simulink model "Powertrain_Performance_Design"  (R2024a)
settings: Solver=ode4  StartTime=0.0  StopTime=simtime  FixedStep=1  MaxStep=0.1  RelTol=1e-3
model workspace (MAT data in the model file):
  A_max = 2.22
  C_d = 0.23
  C_r = 0.011
  Cpack = 216
  DOD = [0 0.1 0.2 0.3 0.4 0.5 0.6 0.7 0.8 0.9 1 1.1 ... (1001 elements, 1001x1)]
  EM_N = [0 100 200 300 400 500 600 700 800 900 1000 1100 1200 1300 1400 1500 1600 1700 1800 1900 2000 2100 2200 2300 2400 2500 2600 2700 2800 2900 3000 3100 3200 3300 3400 3500 3600 3700 3800 3900 4000 4100 4200 4300 4400 4500 4600 4700 4800 4900 5000 5100 5200 5300 5400 5500 5600 5700 5800 5900 6000 6100 6200 6300 6400 6500 6600 6700 6800 6900 7000 7100 7200 7300 7400 7500 7600 7700 7800 7900 8000 8100 8200 8300 8400 8500 8600 8700 8800 8900 9000 9100 9200 9300 9400 9500 9600 9700 9800 9900 10000 10100 10200 10300 10400 10500 10600 10700 10800 10900 11000 11100 11200 11300 11400 11500 11600 11700 11800 11900 12000 12100 12200 12300 12400 12500 12600 12700 12800 12900 13000 13100 13200 13300 13400 13500 13600 13700 13800 13900 14000 14100 14200 14300 14400 14500 14600 14700 14800 14900 15000 15100 15200 15300 15400 15500 15600 15700 15800 15900 16000 16100 16200 16300 16400 16500 16600 16700 16800 16900 17000]
  EM_N_Max = 17000
  EM_N_Min = 0
  EM_eff = Simulink.Parameter
  EM_eff.Value = [78 78 78 78 78 78 78 78 78 78 78 78 ... (250000 elements, 500x500)]
  EM_eff.Complexity = 'real'
  EM_eff.Dimensions = [500 500]
  EM_eff.DataType = 'auto'
  Ff_N = 10218
  Kd = 0.3
  Ki = 0.02
  Kp = 15
  N_EM_eff = [0 34.06813627 68.13627255 102.2044088 136.2725451 170.3406814 204.4088176 238.4769539 272.5450902 306.6132265 340.6813627 374.749499 ... (500 elements, 1x500)]
  T_EM_Cont = [181.43664; 181.43664; 181.43664; 181.43664; 181.43664; 181.43664; 181.43664; 181.43664; 181.43664; 181.43664; 181.43664; 181.43664; 181.43664; 181.43664; 181.43664; 181.43664; 181.43664; 181.43664; 181.43664; 181.43664; 181.43664; 181.43664; 181.43664; 181.43664; 181.43664; 181.43664; 181.43664; 181.43664; 181.43664; 181.43664; 181.43664; 181.43664; 181.43664; 181.43664; 181.43664; 181.43664; 181.43664; 181.43664; 181.43664; 181.43664; 181.43664; 181.43664; 181.43664; 181.43664; 181.43664; 181.43664; 181.43664; 181.43664; 181.43664; 181.43664; 181.43664; 177.87905; 174.4583; 171.16664; 167.99688; 164.9424; 161.997; 159.15494; 156.41089; 153.75986; 151.1972; 148.71855; 146.31987; 143.99733; 141.74737; 139.56664; 137.452; 135.40047; 133.40929; 131.47582; 129.5976; 127.77228; 125.99766; 124.27167; 122.59232; 120.95776; 119.36621; 117.816; 116.30554; 114.83331; 113.3979; 111.99792; 110.63209; 109.29918; 107.998; 106.72743; 105.48642; 104.27393; 103.089; 101.93069; 100.79813; 99.690459; 98.606867; 97.546578; 96.508848; 95.492966; 94.498247; 93.524039; 92.569712; 91.634664; 90.718318; 89.820116; 88.939527; 88.076036; 87.229152; 86.398398; 85.583318; 84.783474; 83.998442; 83.227814; 82.471198; 81.728214; 80.998498; 80.281697; 79.577472; 78.885494; 78.205446; 77.537024; 76.87993; 76.23388; 75.598598; 74.973816; 74.359277; 73.75473; 73.159934; 72.574654; 71.998665; 71.431746; 70.873686; 70.324277; 69.783321; 69.250624; 68.725998; 68.209261; 67.700237; 67.198754; 66.704645; 66.21775; 65.737911; 65.264977; 64.798798; 64.339232; 63.886139; 63.439383; 62.998832; 62.564357; 62.135834; 61.713141; 61.296161; 60.884777; 60.478878; 60.078356; 59.683104; 59.293018; 58.907998; 58.527947; 58.152768; 57.782368; 57.416657; 57.055546; 56.698948; 56.346781; 55.998961; 55.65541; 55.316047; 54.980799; 54.649589; 54.322346; 53.998999; 53.679478; 53.363716]
  T_EM_Max = 375
  T_EM_Min = -375
  T_EM_Peak = [375; 375; 375; 375; 375; 375; 375; 375; 375; 375; 375; 375; 375; 375; 375; 375; 375; 375; 375; 375; 375; 375; 375; 375; 375; 375; 375; 375; 375; 375; 375; 375; 375; 375; 375; 375; 375; 375; 375; 375; 375; 375; 375; 375; 375; 375; 375; 375; 375; 375; 375; 368.86499; 361.77143; 354.94555; 348.37249; 342.03844; 335.93061; 330.03709; 324.3468; 318.84939; 313.53524; 308.39532; 303.4212; 298.60499; 293.93929; 289.41714; 285.03203; 280.77782; 276.64874; 272.63934; 268.74449; 264.95936; 261.27936; 257.7002; 254.21776; 250.82819; 247.52782; 244.31317; 241.18095; 238.12803; 235.15143; 232.24832; 229.41603; 226.65198; 223.95374; 221.31899; 218.74551; 216.2312; 213.77403; 211.37207; 209.02349; 206.72653; 204.4795; 202.2808; 200.12888; 198.02226; 195.95952; 193.93932; 191.96035; 190.02136; 188.12114; 186.25856; 184.43249; 182.64189; 180.88571; 179.16299; 177.47278; 175.81415; 174.18624; 172.5882; 171.01922; 169.47851; 167.96531; 166.47889; 165.01855; 163.5836; 162.1734; 160.7873; 159.4247; 158.08499; 156.76762; 155.47202; 154.19766; 152.94402; 151.7106; 150.49691; 149.30249; 148.12688; 146.96964; 145.83034; 144.70857; 143.60393; 142.51602; 141.44447; 140.38891; 139.34899; 138.32437; 137.3147; 136.31967; 135.33895; 134.37224; 133.41925; 132.47968; 131.55325; 130.63968; 129.73872; 128.8501; 127.97357; 127.10888; 126.2558; 125.4141; 124.58354; 123.76391; 122.955; 122.15659; 121.36848; 120.59048; 119.82238; 119.06401; 118.31518; 117.57571; 116.84543; 116.12416; 115.41174; 114.70801; 114.01281; 113.32599; 112.64739; 111.97687; 111.31429; 110.6595]
  Tq_EM_eff = [0 0.751503006 1.503006012 2.254509018 3.006012024 3.75751503 4.509018036 5.260521042 6.012024048 6.763527054 7.51503006 8.266533066 ... (500 elements, 1x500)]
  Upack = [405.9 404.506 403.17334 401.89932 400.68136 399.51699 398.40386 397.33971 396.32239 395.34983 394.42006 393.53121 ... (1001 elements, 1001x1)]
  Upack_max = 405.9
  Vmax = 250
  a_r = 1.202
  eta_pack = 0.97
  eta_tr = 0.95
  g = 9.81
  ix = 9
  lambda_m = 1.05
  m_v = 1862
  r_w = 0.3277
  t_cool = 250
  t_peak = 20
values from neighbouring files (symbols this model uses):
  EM_eff = [78 78 78 78 78 78 78 78 78 78 78 78 ... (250000 elements, 500x500)]    [EM_eff.mat]
undefined symbols (not defined in the file or in its folder): selection, Soc_init, theta
(part 1 of 2)
settings Model: Creator=Kimo Store  LastModifiedBy=Kimo Store
settings DataIOCC: SaveOutput=off  ReturnWorkspaceOutputs=off  LoggingToFile=on
settings ConfigComp: DVTestSuiteOptimization=Auto  DVDetectOutOfBounds=on  DVModelReferenceHarness=on  DVHarnessSource=Signal Editor

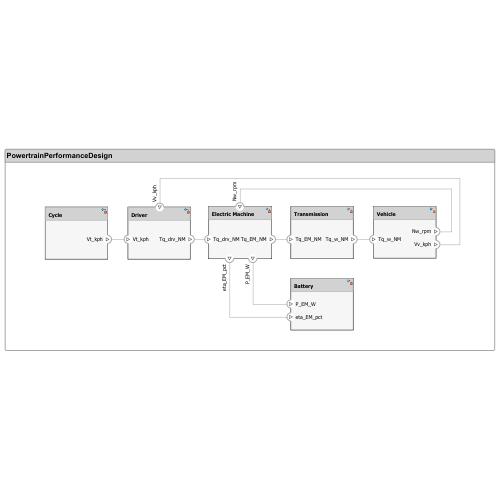
[thumbnail: Simulink's stored preview of the top-level diagram]
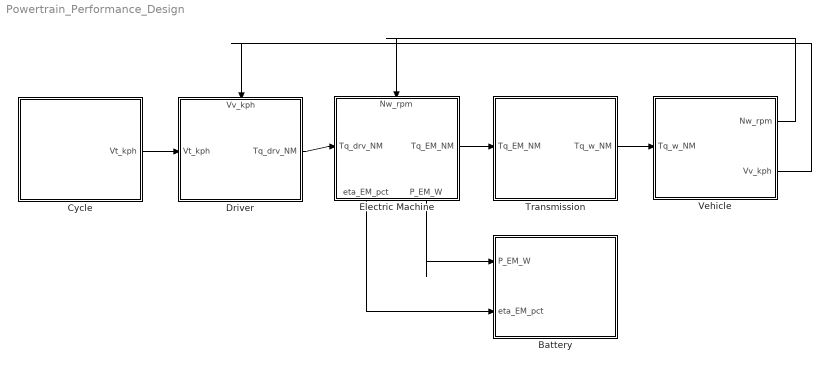
== system Powertrain_Performance_Design ==
  Battery : Subsystem
      settings: PortSchema="{\"entries\":[{\"content\":{\"headerSize\":26,\"margin\":15,\"minimumSpacing\":25,\"sides\":[{\"content\":{\"connectorIds\":[\"In1\",\"In2\"]},\"type\":\"ConnectorPlacement.EquallySpacedRectSide\",\"uuid\":\"68db000f-08f3-43d6-8df8-ef1e265f9696\"},{\"content\":{\"side\":\"RIGHT\"},\"type\":\"ConnectorPlacement.EquallySpacedRectSide\",\"uuid\":\"83cc5010-d255-45a5-b8a1-63c53c107bd8\"},{\"content\":{\"side\":\"TOP\"},\"type\":\"ConnectorPlacement.EquallySpacedRectSide\",\"uuid\":\"8183809d-813b-433e-980f-1f031c5b719a\"}]},\"type\":\"ConnectorPlacement.EquallySpacedConnector\",\"uuid\":\"7d483e94-2e91-4ff8-9657-91e4b1686e41\"}],\"packageUris\":[\"http://schema.mathworks.com/mf0/Connector/R2020b\"],\"version\":\"1.0\"}"
  Cycle : Subsystem
      settings: PortSchema="{\"entries\":[{\"content\":{\"headerSize\":26,\"margin\":15,\"minimumSpacing\":25,\"sides\":[{\"content\":{},\"type\":\"ConnectorPlacement.EquallySpacedRectSide\",\"uuid\":\"68db000f-08f3-43d6-8df8-ef1e265f9696\"},{\"content\":{\"connectorIds\":[\"Out1\"],\"side\":\"RIGHT\"},\"type\":\"ConnectorPlacement.EquallySpacedRectSide\",\"uuid\":\"83cc5010-d255-45a5-b8a1-63c53c107bd8\"},{\"content\":{\"side\":\"TOP\"},\"type\":\"ConnectorPlacement.EquallySpacedRectSide\",\"uuid\":\"8183809d-813b-433e-980f-1f031c5b719a\"}]},\"type\":\"ConnectorPlacement.EquallySpacedConnector\",\"uuid\":\"7d483e94-2e91-4ff8-9657-91e4b1686e41\"}],\"packageUris\":[\"http://schema.mathworks.com/mf0/Connector/R2020b\"],\"version\":\"1.0\"}"
  Driver : Subsystem
      settings: PortSchema="{\"entries\":[{\"content\":{\"headerSize\":26,\"margin\":15,\"minimumSpacing\":25,\"sides\":[{\"content\":{\"connectorIds\":[\"In2\"]},\"type\":\"ConnectorPlacement.EquallySpacedRectSide\",\"uuid\":\"68db000f-08f3-43d6-8df8-ef1e265f9696\"},{\"content\":{\"connectorIds\":[\"Out1\"],\"side\":\"RIGHT\"},\"type\":\"ConnectorPlacement.EquallySpacedRectSide\",\"uuid\":\"83cc5010-d255-45a5-b8a1-63c53c107bd8\"},{\"content\":{\"connectorIds\":[\"In1\"],\"side\":\"TOP\"},\"type\":\"ConnectorPlacement.EquallySpacedRectSide\",\"uuid\":\"8183809d-813b-433e-980f-1f031c5b719a\"}]},\"type\":\"ConnectorPlacement.EquallySpacedConnector\",\"uuid\":\"7d483e94-2e91-4ff8-9657-91e4b1686e41\"}],\"packageUris\":[\"http://schema.mathworks.com/mf0/Connector/R2020b\"],\"version\":\"1.0\"}"
  Electric Machine : Subsystem
      settings: PortSchema="{\"entries\":[{\"content\":{\"headerSize\":26,\"margin\":15,\"minimumSpacing\":25,\"sides\":[{\"content\":{\"connectorIds\":[\"In2\"]},\"type\":\"ConnectorPlacement.EquallySpacedRectSide\",\"uuid\":\"68db000f-08f3-43d6-8df8-ef1e265f9696\"},{\"content\":{\"connectorIds\":[\"Out1\"],\"side\":\"RIGHT\"},\"type\":\"ConnectorPlacement.EquallySpacedRectSide\",\"uuid\":\"83cc5010-d255-45a5-b8a1-63c53c107bd8\"},{\"content\":{\"connectorIds\":[\"In1\"],\"side\":\"TOP\"},\"type\":\"ConnectorPlacement.EquallySpacedRectSide\",\"uuid\":\"8183809d-813b-433e-980f-1f031c5b719a\"},{\"content\":{\"connectorIds\":[\"Out3\",\"Out2\"],\"side\":\"BOTTOM\"},\"type\":\"ConnectorPlacement.EquallySpacedRectSide\",\"uuid\":\"47240857-0798-46c4-9ad5-1efcb742b832\"}]},\"type\":\"ConnectorPlacement.EquallySpacedConnector\",\"uuid\":\"7d483e94-2e91-4ff8-9657-91e4b1686e41\"}],\"packageUris\":[\"http://schema.mathworks.com/mf0/Connector/R2020b\"],\"version\":\"1.0\"}"
  Transmission : Subsystem
      settings: PortSchema="{\"entries\":[{\"content\":{\"headerSize\":26,\"margin\":15,\"minimumSpacing\":25,\"sides\":[{\"content\":{\"connectorIds\":[\"In1\"]},\"type\":\"ConnectorPlacement.EquallySpacedRectSide\",\"uuid\":\"68db000f-08f3-43d6-8df8-ef1e265f9696\"},{\"content\":{\"connectorIds\":[\"Out1\"],\"side\":\"RIGHT\"},\"type\":\"ConnectorPlacement.EquallySpacedRectSide\",\"uuid\":\"83cc5010-d255-45a5-b8a1-63c53c107bd8\"},{\"content\":{\"side\":\"TOP\"},\"type\":\"ConnectorPlacement.EquallySpacedRectSide\",\"uuid\":\"8183809d-813b-433e-980f-1f031c5b719a\"}]},\"type\":\"ConnectorPlacement.EquallySpacedConnector\",\"uuid\":\"7d483e94-2e91-4ff8-9657-91e4b1686e41\"}],\"packageUris\":[\"http://schema.mathworks.com/mf0/Connector/R2020b\"],\"version\":\"1.0\"}"
  Vehicle : Subsystem
      settings: PortSchema="{\"entries\":[{\"content\":{\"headerSize\":26,\"margin\":15,\"minimumSpacing\":25,\"sides\":[{\"content\":{\"connectorIds\":[\"In1\"]},\"type\":\"ConnectorPlacement.EquallySpacedRectSide\",\"uuid\":\"68db000f-08f3-43d6-8df8-ef1e265f9696\"},{\"content\":{\"connectorIds\":[\"Out1\",\"Out2\"],\"side\":\"RIGHT\"},\"type\":\"ConnectorPlacement.EquallySpacedRectSide\",\"uuid\":\"83cc5010-d255-45a5-b8a1-63c53c107bd8\"},{\"content\":{\"side\":\"TOP\"},\"type\":\"ConnectorPlacement.EquallySpacedRectSide\",\"uuid\":\"8183809d-813b-433e-980f-1f031c5b719a\"},{\"content\":{\"side\":\"BOTTOM\"},\"type\":\"ConnectorPlacement.EquallySpacedRectSide\",\"uuid\":\"d8f33a88-2120-49d7-a1ee-2682923ccda4\"}]},\"type\":\"ConnectorPlacement.EquallySpacedConnector\",\"uuid\":\"7d483e94-2e91-4ff8-9657-91e4b1686e41\"}],\"packageUris\":[\"http://schema.mathworks.com/mf0/Connector/R2020b\"],\"version\":\"1.0\"}"
  wires:
  Electric Machine/2(P_EM_W) -> Battery/1(P_EM_W)
  Driver/1(Tq_drv_NM) -> Electric Machine/2(Tq_drv_NM)
  Vehicle/1(Nw_rpm) -> Electric Machine/1(Nw_rpm)
  Transmission/1(Tq_w_NM) -> Vehicle/1(Tq_w_NM)
  Electric Machine/3(eta_EM_pct) -> Battery/2(eta_EM_pct)
  Electric Machine/1(Tq_EM_NM) -> Transmission/1(Tq_EM_NM)
  Vehicle/2(Vv_kph) -> Driver/1(Vv_kph)
  Cycle/1(Vt_kph) -> Driver/2(Vt_kph)

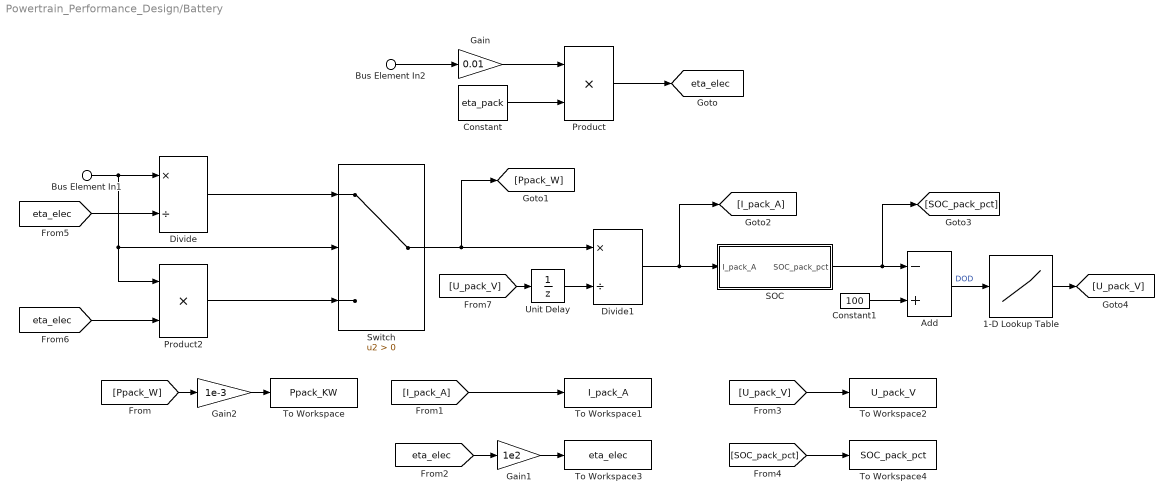
== system Powertrain_Performance_Design/Battery ==
  Bus Element In1 : Inport  PortName=P_EM_W
  Bus Element In2 : Inport  Port=2  PortName=eta_EM_pct
  1-D Lookup Table : Lookup_n-D  NumberOfTableDimensions=1  BreakpointsForDimension1=DOD  Table=Upack  InternalRulePriority=Speed  RndMeth=Simplest
  Add : Sum  Inputs=-+
  Constant : Constant  Value=eta_pack
  Constant1 : Constant  Value=100
  Divide : Product  Inputs=*/
  Divide1 : Product  Inputs=*/
  Gain : Gain  Gain=0.01
  Gain1 : Gain  Gain=1e2
  Gain2 : Gain  Gain=1e-3
  Product : Product
  Product2 : Product
  SOC : Subsystem
  Switch : Switch  Criteria=u2 > Threshold  SaturateOnIntegerOverflow=off  InputSameDT=off
  To Workspace : ToWorkspace  VariableName=Ppack_KW  SaveFormat=Timeseries  SampleTime=-1
  To Workspace1 : ToWorkspace  VariableName=I_pack_A  SaveFormat=Timeseries  SampleTime=-1
  To Workspace2 : ToWorkspace  VariableName=U_pack_V  SaveFormat=Timeseries  SampleTime=-1
  To Workspace3 : ToWorkspace  VariableName=eta_elec  SaveFormat=Timeseries  SampleTime=-1
  To Workspace4 : ToWorkspace  VariableName=SOC_pack_pct  SaveFormat=Timeseries  SampleTime=-1
  Unit Delay : UnitDelay  InitialCondition=405.9  SampleTime=-1  HasFrameUpgradeWarning=on
  tag scope: eta_elec=global
  wires:
  Bus Element In2/1 -> Gain/1
  Gain/1 -> Product/1
  Constant/1 -> Product/2
  Product/1 -> [eta_elec]
  [Ppack_W] -> Gain2/1
  [I_pack_A] -> To Workspace1/1
  [U_pack_V] -> To Workspace2/1
  [SOC_pack_pct] -> To Workspace4/1
  [eta_elec] -> Gain1/1
  Gain1/1 -> To Workspace3/1
  Divide/1 -> Switch/1
  Product2/1 -> Switch/3
  Switch/1 -> Divide1/1, [Ppack_W]
  Bus Element In1/1 -> Switch/2, Product2/1, Divide/1
  [eta_elec] -> Divide/2
  [eta_elec] -> Product2/2
  Divide1/1 -> [I_pack_A], SOC/1(I_pack_A)
  SOC/1(SOC_pack_pct) -> [SOC_pack_pct], Add/1
  Constant1/1 -> Add/2
  Unit Delay/1 -> Divide1/2
  [U_pack_V] -> Unit Delay/1
  Add/1 -> 1-D Lookup Table/1  "DOD"
  1-D Lookup Table/1 -> [U_pack_V]
  Gain2/1 -> To Workspace/1

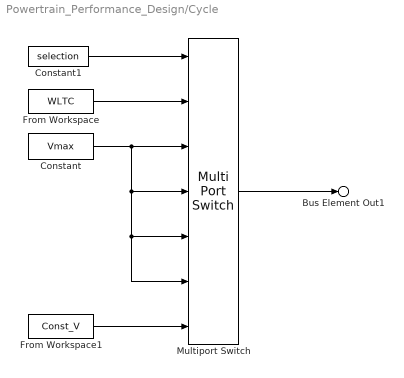
== system Powertrain_Performance_Design/Cycle ==
  Constant : Constant  Value=Vmax
  Constant1 : Constant  Value=selection
  From Workspace : FromWorkspace  VariableName=WLTC
  From Workspace1 : FromWorkspace  VariableName=Const_V
  Multiport Switch : MultiPortSwitch  Inputs=6  SaturateOnIntegerOverflow=off  InputSameDT=off
  Bus Element Out1 : Outport  PortName=Vt_kph
  wires:
  Multiport Switch/1 -> Bus Element Out1/1
  From Workspace/1 -> Multiport Switch/2
  Constant/1 -> Multiport Switch/5, Multiport Switch/6, Multiport Switch/4, Multiport Switch/3
  Constant1/1 -> Multiport Switch/1
  From Workspace1/1 -> Multiport Switch/7

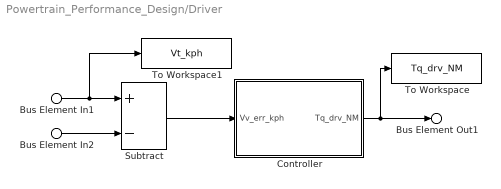
== system Powertrain_Performance_Design/Driver ==
  Bus Element In2 : Inport  PortName=Vv_kph
  Bus Element In1 : Inport  Port=2  PortName=Vt_kph
  Controller : Subsystem
  Subtract : Sum  Inputs=+-
  To Workspace : ToWorkspace  VariableName=Tq_drv_NM  SaveFormat=Timeseries  SampleTime=-1
  To Workspace1 : ToWorkspace  VariableName=Vt_kph  SaveFormat=Timeseries  SampleTime=-1
  Bus Element Out1 : Outport  PortName=Tq_drv_NM
  wires:
  Bus Element In1/1 -> To Workspace1/1, Subtract/1
  Bus Element In2/1 -> Subtract/2
  Subtract/1 -> Controller/1(Vv_err_kph)
  Controller/1(Tq_drv_NM) -> To Workspace/1, Bus Element Out1/1

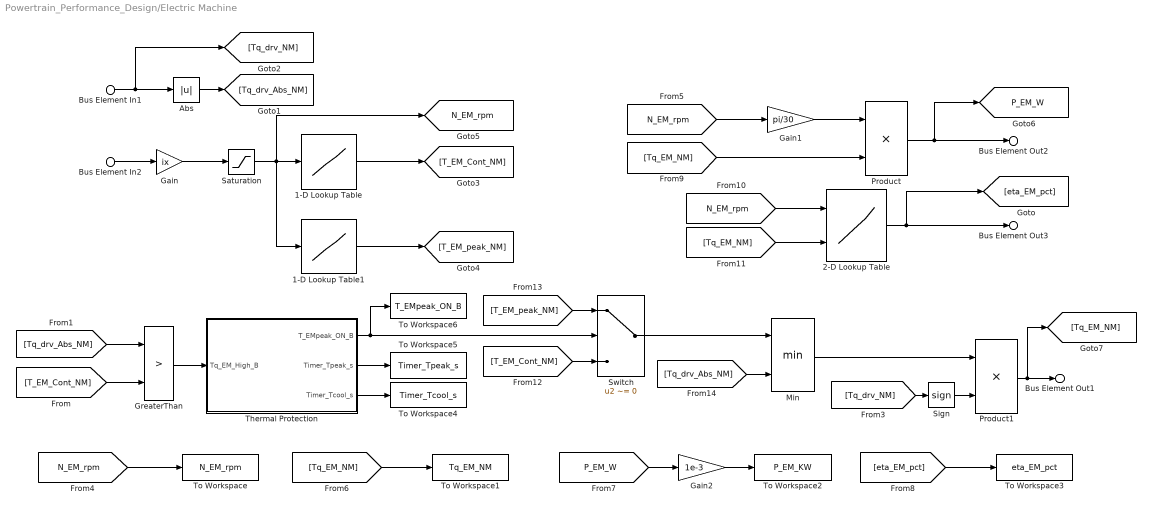
== system Powertrain_Performance_Design/Electric Machine ==
  Bus Element In2 : Inport  PortName=Nw_rpm
  Bus Element In1 : Inport  Port=2  PortName=Tq_drv_NM
  1-D Lookup Table : Lookup_n-D  NumberOfTableDimensions=1  BreakpointsForDimension1=EM_N  Table=T_EM_Cont  InternalRulePriority=Speed  RndMeth=Simplest
  1-D Lookup Table1 : Lookup_n-D  NumberOfTableDimensions=1  BreakpointsForDimension1=EM_N  Table=T_EM_Peak  InternalRulePriority=Speed  RndMeth=Simplest
  2-D Lookup Table : Lookup_n-D  BreakpointsForDimension1=N_EM_eff  BreakpointsForDimension2=Tq_EM_eff  Table=EM_eff  InternalRulePriority=Speed  RndMeth=Simplest
      settings: InputPortMap=u0,u1
  Abs : Abs  SaturateOnIntegerOverflow=off
  Gain : Gain  Gain=ix
  Gain1 : Gain  Gain=pi/30
  Gain2 : Gain  Gain=1e-3
  GreaterThan : RelationalOperator  Operator=>  OutDataTypeStr=boolean  RndMeth=Simplest  InputSameDT=off
  Min : MinMax  Inputs=2
  Product : Product
  Product1 : Product
  Saturation : Saturate  UpperLimit=EM_N_Max  LowerLimit=EM_N_Min
  Sign : Signum
  Switch : Switch  Criteria=u2 ~= 0  SaturateOnIntegerOverflow=off  InputSameDT=off
  Thermal Protection : Subsystem
  To Workspace : ToWorkspace  VariableName=N_EM_rpm  SaveFormat=Timeseries  SampleTime=-1
  To Workspace1 : ToWorkspace  VariableName=Tq_EM_NM  SaveFormat=Timeseries  SampleTime=-1
  To Workspace2 : ToWorkspace  VariableName=P_EM_KW  SaveFormat=Timeseries  SampleTime=-1
  To Workspace3 : ToWorkspace  VariableName=eta_EM_pct  SaveFormat=Timeseries  SampleTime=-1
  To Workspace4 : ToWorkspace  VariableName=Timer_Tcool_s  SaveFormat=Timeseries  SampleTime=-1
  To Workspace5 : ToWorkspace  VariableName=Timer_Tpeak_s  SaveFormat=Timeseries  SampleTime=-1
  To Workspace6 : ToWorkspace  VariableName=T_EMpeak_ON_B  SaveFormat=Timeseries  SampleTime=-1
  Bus Element Out1 : Outport  PortName=Tq_EM_NM
  Bus Element Out2 : Outport  Port=2  PortName=P_EM_W
  Bus Element Out3 : Outport  Port=3  PortName=eta_EM_pct
  tag scope: N_EM_rpm=global, P_EM_W=global
  wires:
  Bus Element In2/1 -> Gain/1
  Gain/1 -> Saturation/1
  Bus Element In1/1 -> Abs/1, [Tq_drv_NM]
  Abs/1 -> [Tq_drv_Abs_NM]
  Saturation/1 -> [N_EM_rpm], 1-D Lookup Table1/1, 1-D Lookup Table/1
  1-D Lookup Table/1 -> [T_EM_Cont_NM]
  1-D Lookup Table1/1 -> [T_EM_peak_NM]
  [N_EM_rpm] -> To Workspace/1
  [N_EM_rpm] -> Gain1/1
  Gain1/1 -> Product/1
  [Tq_EM_NM] -> To Workspace1/1
  Gain2/1 -> To Workspace2/1
  [P_EM_W] -> Gain2/1
  [eta_EM_pct] -> To Workspace3/1
  [Tq_EM_NM] -> Product/2
  2-D Lookup Table/1 -> [eta_EM_pct], Bus Element Out3/1
  [N_EM_rpm] -> 2-D Lookup Table/1
  [Tq_EM_NM] -> 2-D Lookup Table/2
  GreaterThan/1 -> Thermal Protection/1(Tq_EM_High_B)
  [T_EM_Cont_NM] -> GreaterThan/2
  [Tq_drv_Abs_NM] -> GreaterThan/1
  Thermal Protection/2(Timer_Tpeak_s) -> To Workspace5/1
  Thermal Protection/1(T_EMpeak_ON_B) -> To Workspace6/1, Switch/2
  Switch/1 -> Min/1
  [Tq_drv_Abs_NM] -> Min/2
  Min/1 -> Product1/1
  Sign/1 -> Product1/2
  [Tq_drv_NM] -> Sign/1
  Product1/1 -> [Tq_EM_NM], Bus Element Out1/1
  Product/1 -> [P_EM_W], Bus Element Out2/1
  Thermal Protection/3(Timer_Tcool_s) -> To Workspace4/1
  [T_EM_Cont_NM] -> Switch/3
  [T_EM_peak_NM] -> Switch/1

== system Powertrain_Performance_Design/Transmission ==
  Bus Element In1 : Inport  PortName=Tq_EM_NM
  Gain : Gain  Gain=eta_tr
  Gain1 : Gain  Gain=ix
  To Workspace : ToWorkspace  VariableName=Tq_w_NM  SaveFormat=Timeseries  SampleTime=-1
  Bus Element Out1 : Outport  PortName=Tq_w_NM
  wires:
  Gain1/1 -> Gain/1
  Gain/1 -> To Workspace/1, Bus Element Out1/1
  Bus Element In1/1 -> Gain1/1

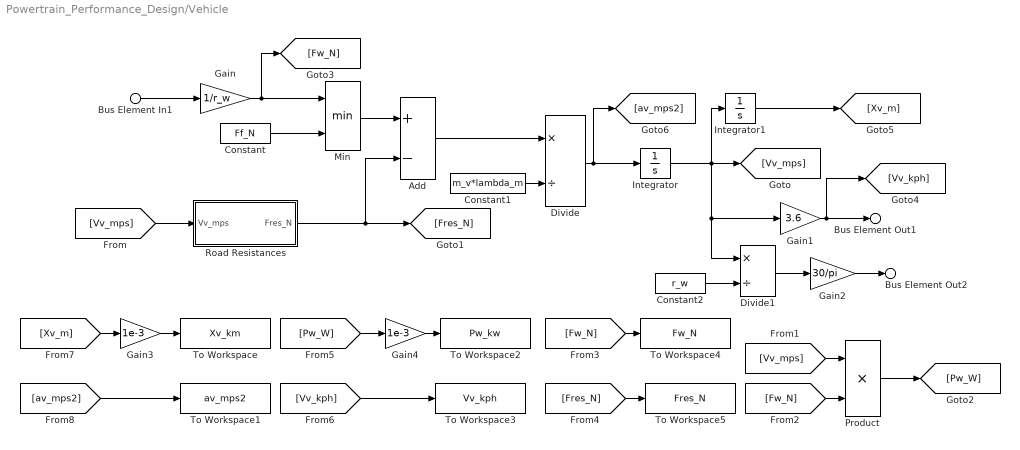
== system Powertrain_Performance_Design/Vehicle ==
  Bus Element In1 : Inport  PortName=Tq_w_NM
  Add : Sum  Inputs=+-
  Constant : Constant  Value=Ff_N
  Constant1 : Constant  Value=m_v*lambda_m
  Constant2 : Constant  Value=r_w
  Divide : Product  Inputs=*/
  Divide1 : Product  Inputs=*/
  Gain : Gain  Gain=1/r_w
  Gain1 : Gain  Gain=3.6
  Gain2 : Gain  Gain=30/pi
  Gain3 : Gain  Gain=1e-3
  Gain4 : Gain  Gain=1e-3
  Integrator : Integrator  UpperSaturationLimit=70  LowerSaturationLimit=0
  Integrator1 : Integrator
  Min : MinMax  Inputs=2
  Product : Product
  Road Resistances : Subsystem
  To Workspace : ToWorkspace  VariableName=Xv_km  SaveFormat=Timeseries  SampleTime=-1
  To Workspace1 : ToWorkspace  VariableName=av_mps2  SaveFormat=Timeseries  SampleTime=-1
  To Workspace2 : ToWorkspace  VariableName=Pw_kw  SaveFormat=Timeseries  SampleTime=-1
  To Workspace3 : ToWorkspace  VariableName=Vv_kph  SaveFormat=Timeseries  SampleTime=-1
  To Workspace4 : ToWorkspace  VariableName=Fw_N  SaveFormat=Timeseries  SampleTime=-1
  To Workspace5 : ToWorkspace  VariableName=Fres_N  SaveFormat=Timeseries  SampleTime=-1
  Bus Element Out2 : Outport  PortName=Nw_rpm
  Bus Element Out1 : Outport  Port=2  PortName=Vv_kph
  wires:
  Bus Element In1/1 -> Gain/1
  Gain/1 -> Min/1, [Fw_N]
  Min/1 -> Add/1
  Add/1 -> Divide/1
  Divide/1 -> Integrator/1, [av_mps2]
  Gain1/1 -> [Vv_kph], Bus Element Out1/1
  Integrator/1 -> Integrator1/1, [Vv_mps], Divide1/1, Gain1/1
  [Vv_mps] -> Road Resistances/1(Vv_mps)
  Road Resistances/1(Fres_N) -> Add/2, [Fres_N]
  Divide1/1 -> Gain2/1
  Gain2/1 -> Bus Element Out2/1
  Constant2/1 -> Divide1/2
  Product/1 -> [Pw_W]
  [Vv_mps] -> Product/1
  [Fw_N] -> Product/2
  [Fw_N] -> To Workspace4/1
  [Fres_N] -> To Workspace5/1
  [Vv_kph] -> To Workspace3/1
  Integrator1/1 -> [Xv_m]
  [Xv_m] -> Gain3/1
  Gain3/1 -> To Workspace/1
  [av_mps2] -> To Workspace1/1
  Constant1/1 -> Divide/2
  [Pw_W] -> Gain4/1
  Gain4/1 -> To Workspace2/1
  Constant/1 -> Min/2

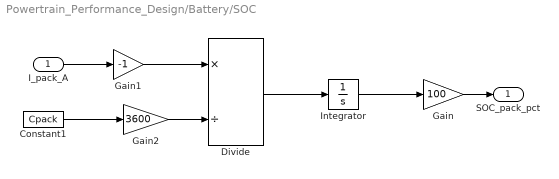
== system Powertrain_Performance_Design/Battery/SOC ==
  I_pack_A : Inport
  Constant1 : Constant  Value=Cpack
  Divide : Product  Inputs=*/
  Gain : Gain  Gain=100
  Gain1 : Gain  Gain=-1
  Gain2 : Gain  Gain=3600
  Integrator : Integrator  InitialCondition=Soc_init  LimitOutput=on  UpperSaturationLimit=1  LowerSaturationLimit=0
  SOC_pack_pct : Outport
  wires:
  Constant1/1 -> Gain2/1
  Gain/1 -> SOC_pack_pct/1
  Integrator/1 -> Gain/1
  I_pack_A/1 -> Gain1/1
  Gain2/1 -> Divide/2
  Divide/1 -> Integrator/1
  Gain1/1 -> Divide/1

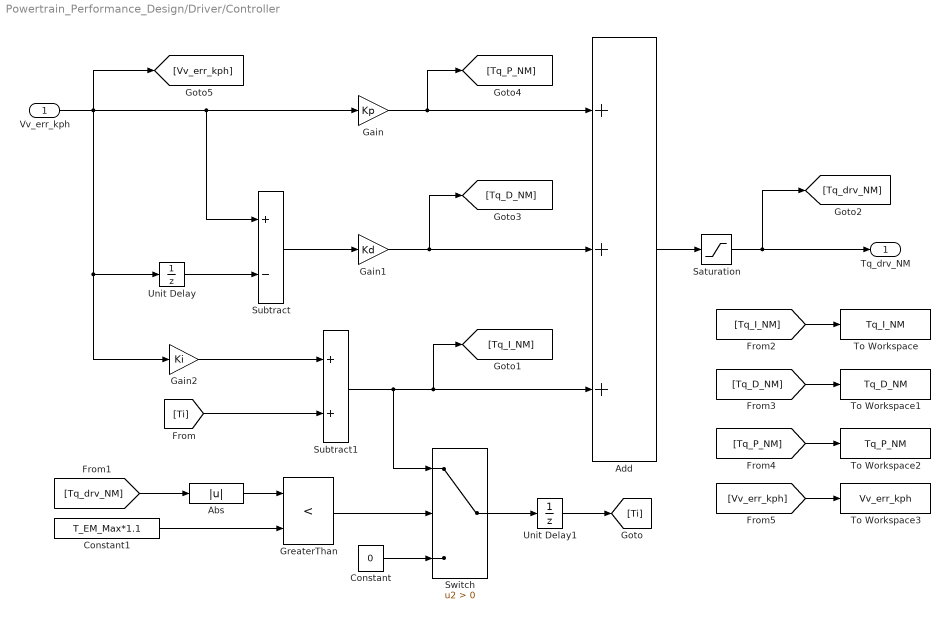
== system Powertrain_Performance_Design/Driver/Controller ==
  Vv_err_kph : Inport
  Abs : Abs  SaturateOnIntegerOverflow=off
  Add : Sum  Inputs=+++
  Constant : Constant  Value=0
  Constant1 : Constant  Value=T_EM_Max*1.1
  Gain : Gain  Gain=Kp
  Gain1 : Gain  Gain=Kd
  Gain2 : Gain  Gain=Ki
  GreaterThan : RelationalOperator  Operator=<  OutDataTypeStr=boolean  RndMeth=Simplest  InputSameDT=off
  Saturation : Saturate  UpperLimit=T_EM_Max*1.1  LowerLimit=T_EM_Min*1.1
  Subtract : Sum  Inputs=+-
  Subtract1 : Sum
  Switch : Switch  Criteria=u2 > Threshold  SaturateOnIntegerOverflow=off  InputSameDT=off
  To Workspace : ToWorkspace  VariableName=Tq_I_NM  SaveFormat=Timeseries  SampleTime=-1
  To Workspace1 : ToWorkspace  VariableName=Tq_D_NM  SaveFormat=Timeseries  SampleTime=-1
  To Workspace2 : ToWorkspace  VariableName=Tq_P_NM  SaveFormat=Timeseries  SampleTime=-1
  To Workspace3 : ToWorkspace  VariableName=Vv_err_kph  SaveFormat=Timeseries  SampleTime=-1
  Unit Delay : UnitDelay  SampleTime=-1  HasFrameUpgradeWarning=on
  Unit Delay1 : UnitDelay  SampleTime=-1  HasFrameUpgradeWarning=on
  Tq_drv_NM : Outport
  wires:
  Add/1 -> Saturation/1
  Gain/1 -> [Tq_P_NM], Add/1
  Vv_err_kph/1 -> [Vv_err_kph], Gain2/1, Unit Delay/1, Subtract/1, Gain/1
  Gain1/1 -> Add/2, [Tq_D_NM]
  Subtract/1 -> Gain1/1
  Unit Delay/1 -> Subtract/2
  Switch/1 -> Unit Delay1/1
  Gain2/1 -> Subtract1/1
  Subtract1/1 -> Switch/1, [Tq_I_NM], Add/3
  Unit Delay1/1 -> [Ti]
  [Ti] -> Subtract1/2
  Constant/1 -> Switch/3
  GreaterThan/1 -> Switch/2
  Constant1/1 -> GreaterThan/2
  Abs/1 -> GreaterThan/1
  [Tq_drv_NM] -> Abs/1
  [Tq_I_NM] -> To Workspace/1
  [Tq_D_NM] -> To Workspace1/1
  [Tq_P_NM] -> To Workspace2/1
  [Vv_err_kph] -> To Workspace3/1
  Saturation/1 -> [Tq_drv_NM], Tq_drv_NM/1

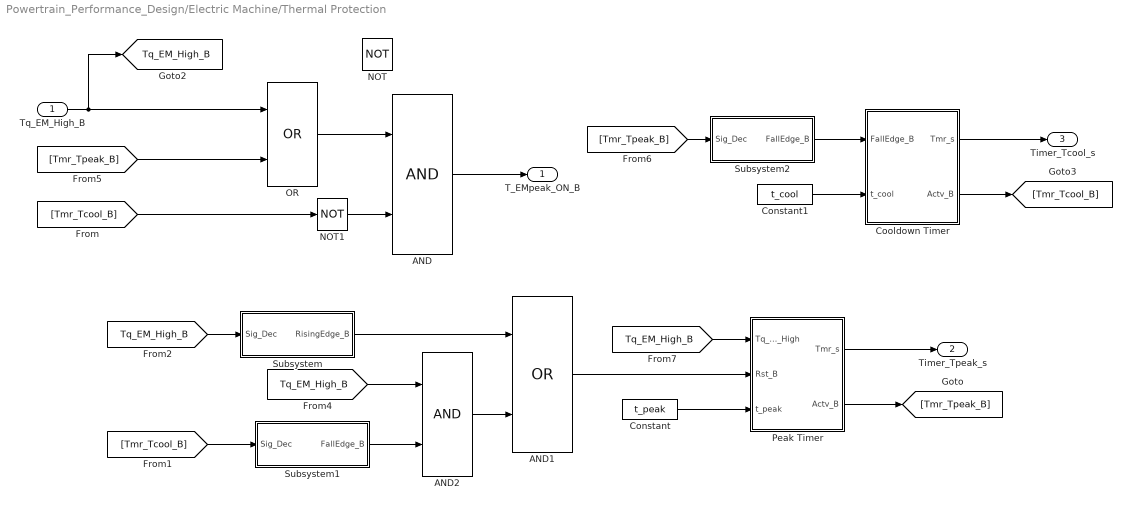
== system Powertrain_Performance_Design/Electric Machine/Thermal Protection ==
  Tq_EM_High_B : Inport
  AND : Logic  AllPortsSameDT=off  OutDataTypeStr=boolean
  AND1 : Logic  Operator=OR  AllPortsSameDT=off  OutDataTypeStr=boolean
  AND2 : Logic  AllPortsSameDT=off  OutDataTypeStr=boolean
  Constant : Constant  Value=t_peak
  Constant1 : Constant  Value=t_cool
  Cooldown Timer : Subsystem
  NOT : Logic  Operator=NOT  IconShape=distinctive  AllPortsSameDT=off  OutDataTypeStr=boolean
  NOT1 : Logic  Operator=NOT  IconShape=distinctive  AllPortsSameDT=off  OutDataTypeStr=boolean
  OR : Logic  Operator=OR  AllPortsSameDT=off  OutDataTypeStr=boolean
  Peak Timer : Subsystem
  Subsystem : Subsystem
  Subsystem1 : Subsystem
  Subsystem2 : Subsystem
  T_EMpeak_ON_B : Outport
  Timer_Tpeak_s : Outport  Port=2
  Timer_Tcool_s : Outport  Port=3
  tag scope: Tq_EM_High_B=global
  wires:
  OR/1 -> AND/1
  AND/1 -> T_EMpeak_ON_B/1
  NOT1/1 -> AND/2
  Peak Timer/2(Actv_B) -> [Tmr_Tpeak_B]
  [Tmr_Tpeak_B] -> OR/2
  Peak Timer/1(Tmr_s) -> Timer_Tpeak_s/1
  Cooldown Timer/1(Tmr_s) -> Timer_Tcool_s/1
  AND1/1 -> Peak Timer/2(Rst_B)
  [Tmr_Tcool_B] -> NOT1/1
  AND2/1 -> AND1/2
  [Tq_EM_High_B] -> AND2/1
  Subsystem/1(RisingEdge_B) -> AND1/1
  [Tq_EM_High_B] -> Subsystem/1(Sig_Dec)
  [Tmr_Tcool_B] -> Subsystem1/1(Sig_Dec)
  Subsystem1/1(FallEdge_B) -> AND2/2
  Subsystem2/1(FallEdge_B) -> Cooldown Timer/1(FallEdge_B)
  [Tmr_Tpeak_B] -> Subsystem2/1(Sig_Dec)
  Cooldown Timer/2(Actv_B) -> [Tmr_Tcool_B]
  Constant/1 -> Peak Timer/3(t_peak)
  Constant1/1 -> Cooldown Timer/2(t_cool)
  [Tq_EM_High_B] -> Peak Timer/1(Tq_EM_High)
  Tq_EM_High_B/1 -> OR/1, [Tq_EM_High_B]
